simulink model "tankiNonLinier"  (R2021b)
settings: Solver=VariableStepAuto  StartTime=0.0  StopTime=50.0  RelTol=1e-3
libraries: simulink x1
settings Model: Creator=Asus  LastModifiedBy=Asus
settings DataIOCC: ExternalInput=getinputstruct(op1)  InitialState=getstatestruct(op1)  LoadExternalInput=on  LoadInitialState=on

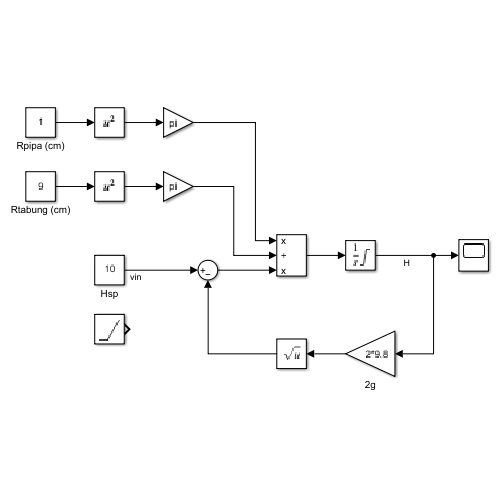
[thumbnail: Simulink's stored preview of the top-level diagram]
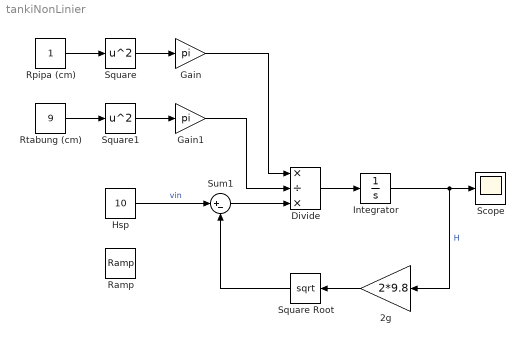
== system tankiNonLinier ==
  2g : Gain  Gain=2*9.8
  Divide : Product  Inputs=*/*
  Gain : Gain  Gain=pi
  Gain1 : Gain  Gain=pi
  Hsp : Constant  Value=10
  Integrator : Integrator  LimitOutput=on  LowerSaturationLimit=0
  Ramp : simulink/Sources/Ramp  slope=1  start=0  InitialOutput=0
  Rpipa (cm) : Constant
  Rtabung (cm) : Constant  Value=9
  Scope : Scope
  Square : Math  Operator=square  SaturateOnIntegerOverflow=on
  Square Root : Sqrt  SaturateOnIntegerOverflow=on
  Square1 : Math  Operator=square  SaturateOnIntegerOverflow=on
  Sum1 : Sum  Inputs=|+-
  wires:
  Integrator/1 -> 2g/1, Scope/1  "H"
  Divide/1 -> Integrator/1
  Sum1/1 -> Divide/3
  2g/1 -> Square Root/1
  Square Root/1 -> Sum1/2
  Rpipa (cm)/1 -> Square/1
  Rtabung (cm)/1 -> Square1/1
  Square1/1 -> Gain1/1
  Square/1 -> Gain/1
  Gain1/1 -> Divide/2
  Gain/1 -> Divide/1
  Hsp/1 -> Sum1/1  "vin"
